simulink model "SM_Regen"  (R2023a)
settings: Solver=ode45  StartTime=0  StopTime=20  FixedStep=0.002  RelTol=1e-3  AbsTol=1e-6
libraries: Solver_SF x1
settings Model: ExtModeTrigMode=oneshot  VariantFading=off  Creator=ywata  LastModifiedBy=USER
settings SolverCC: AutoScaleAbsTol=off  AlgebraicLoopSolver=TrustRegion
settings DataIOCC: SaveFormat=Array  SignalLoggingSaveFormat=ModelDataLogs  ReturnWorkspaceOutputs=off  SignalLoggingName=sigsOut
settings OptimizationCC: BlockReduction=off  BooleanDataType=off  ExpressionDepthLimit=2147483647  LifeSpan=inf
settings DebuggingCC: SaveWithParameterizedLinksMsg=none  UnderspecifiedInitializationDetection=Classic  MergeDetectMultiDrivingBlocksExec=none  SignalResolutionControl=TryResolveAllWithWarning  MultiTaskDSMMsg=warning  MultiTaskCondExecSysMsg=none  FcnCallInpInsideContextMsg=warning  UnconnectedInputMsg=warning  UnconnectedOutputMsg=warning  UnconnectedLineMsg=warning  StateNameClashWarn=warning  SFUnexpectedBacktrackingDiag=warning  SFNoUnconditionalDefaultTransitionDiag=warning  SFExecutionAtInitializationDiag=none  ArithmeticOperatorsInVariantConditions=warning
settings HardwareCC: ProdBitPerPointer=32  ProdBitPerSizeT=32  ProdBitPerPtrDiffT=32  ProdLargestAtomicFloat=None  ProdIntDivRoundTo=Undefined  ProdEndianess=Unspecified  ProdWordSize=32  ProdHWDeviceType=32-bit Generic  TargetUnknown=on
settings ModelReferenceCC: PropagateSignalLabelsOutOfModel=off
settings SFSimCC: SimUseLocalCustomCode=off  CustomCodeUndefinedFunction=UseInterfaceOnly
settings RTWCC: TemplateMakefile=grt_vc.tmf  RTWUseLocalCustomCode=off
settings CodeAppCC: StateflowObjectComments=on
settings GRTTargetCC: TargetFcnLib=ansi_tfl_tmw.mat  TargetLangStandard=C89/C90 (ANSI)  CombineOutputUpdateFcns=off  GRTInterface=on
settings ConfigComp: CovMetricSettings=dw  CovSaveCumulativeToWorkspaceVar=on  CovSaveSingleToWorkspaceVar=on  CovExternalEMLEnable=off

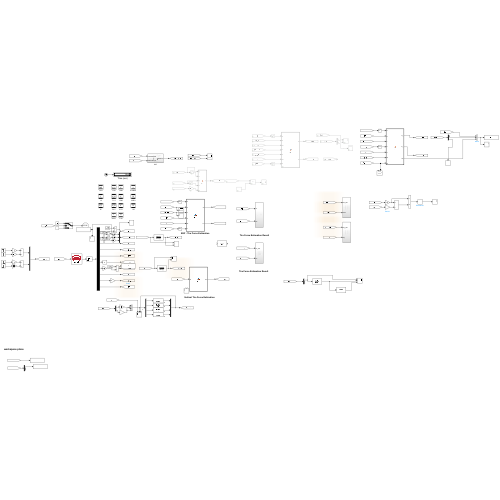
[thumbnail: Simulink's stored preview of the top-level diagram]
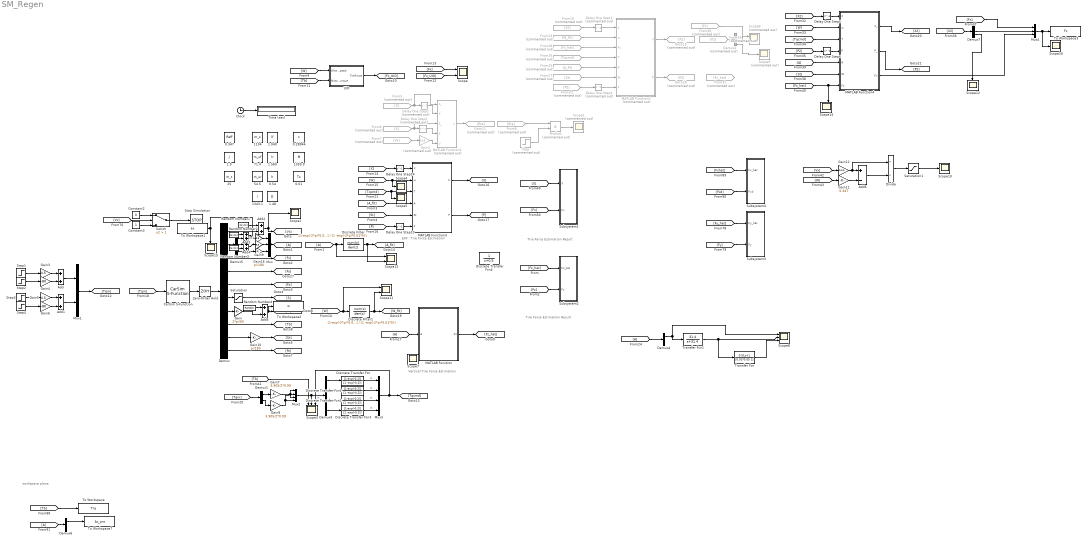
== system SM_Regen ==
  note: workspace place
  note: EKF : Tire Force Estimation
  note: Tire Force Estimation Result
  note: Vertical Tire Force Estimation
  note: Tire Force Estimation Result
  0.01 : DataStoreMemory  DataStoreName=Ts  WriteAfterWriteMsg=warning  InitialValue=0.01  ShowAdditionalParam=off  OutDataTypeStr=double
  0.28944 : DataStoreMemory  DataStoreName=c  WriteAfterWriteMsg=warning  InitialValue=0.29844  ShowAdditionalParam=off  OutDataTypeStr=double
  0.347 : DataStoreMemory  DataStoreName=Reff  WriteAfterWriteMsg=warning  InitialValue=0.347  ShowAdditionalParam=off  OutDataTypeStr=double
  0.54 : DataStoreMemory  DataStoreName=h  WriteAfterWriteMsg=warning  InitialValue=0.54  ShowAdditionalParam=off  OutDataTypeStr=double
  1.040 : DataStoreMemory  DataStoreName=lf  WriteAfterWriteMsg=warning  InitialValue=1.040  ShowAdditionalParam=off  OutDataTypeStr=double
  1.48 : DataStoreMemory  DataStoreName=D  WriteAfterWriteMsg=warning  InitialValue=1.48  ShowAdditionalParam=off  OutDataTypeStr=double
  1.560 : DataStoreMemory  DataStoreName=lr  WriteAfterWriteMsg=warning  InitialValue=1.560  ShowAdditionalParam=off  OutDataTypeStr=double
  1.9 : DataStoreMemory  DataStoreName=J  WriteAfterWriteMsg=warning  InitialValue=1.9  ShowAdditionalParam=off  OutDataTypeStr=double
  1134 : DataStoreMemory  DataStoreName=m_s  WriteAfterWriteMsg=warning  InitialValue=1134  ShowAdditionalParam=off  OutDataTypeStr=double
  1343.1 : DataStoreMemory  DataStoreName=I  WriteAfterWriteMsg=warning  InitialValue=1343.1  ShowAdditionalParam=off  OutDataTypeStr=double
  1359.9 : DataStoreMemory  DataStoreName=M  WriteAfterWriteMsg=warning  InitialValue=1359.9  ShowAdditionalParam=off  OutDataTypeStr=double
  25 : DataStoreMemory  DataStoreName=m_t  WriteAfterWriteMsg=warning  InitialValue=25  ShowAdditionalParam=off  OutDataTypeStr=double
  54.5 : DataStoreMemory  DataStoreName=m_ur  WriteAfterWriteMsg=warning  InitialValue=54.5  ShowAdditionalParam=off  OutDataTypeStr=double
  71.4 : DataStoreMemory  DataStoreName=m_uf  WriteAfterWriteMsg=warning  InitialValue=71.4  ShowAdditionalParam=off  OutDataTypeStr=double
  Add{,1..5} (6 alike) : Sum
  Add6 : Sum  Inputs=+-
  CarSim S-Function : Solver_SF/CarSim S-Function  Priority=1  SIMFILE=simfile.sim  Run_RTs=off  vs_state_ind=Run  StopMode_ind=Vehicle Model
  Clock : Clock
  Constant2 : Constant  Value=0
  Constant3 : Constant
  Delay One Step1 : Delay  Commented=on  DelayLength=1  InitialCondition=[67.655 67.655 67.655 67.655 0 0 0 0 0 0]'  SampleTime=0.01
  Delay One Step10 : Delay  DelayLength=1  InitialCondition=diag([64.1 64.1 64.1 64.1 0 0 0 0])  SampleTime=0.01
  Delay One Step14 : Delay  DelayLength=1  InitialCondition=[64.1 64.1 64.1 64.1 0 0 0 0]'  SampleTime=0.01
  Delay One Step2 : Delay  Commented=on  DelayLength=1  InitialCondition=[0 0 0 0]'  SampleTime=0.01
  Delay One Step3 : Delay  Commented=on  DelayLength=1  InitialCondition=[64.1 64.1 64.1 64.1 0 0 0 0 3930 2740 3930 2740 0]'  SampleTime=0.01
  Delay One Step4 : Delay  Commented=on  DelayLength=1  InitialCondition=diag([64.1 64.1 64.1 64.1 0 0 0 0 3930 2740 3930 2740 0])  SampleTime=0.01
  Delay One Step5 : Delay  DelayLength=1  InitialCondition=[64.1 64.1 64.1 64.1 0 0 0 0 0]'  SampleTime=0.01
  Delay One Step6 : Delay  DelayLength=1  InitialCondition=diag([64.1 64.1 64.1 64.1 0 0 0 0 0])  SampleTime=0.01
  Demux : Demux  Outputs=[1 3 4 4 4 4 4 4 2 2]
  Demux1 : Demux  Outputs=2
  Demux2 : Demux  Commented=on  Outputs=[4 4 4 1]
  Demux3 : Demux
  Demux4 : Demux  Outputs=3
  Demux5 : Demux  Outputs=[1 1 1]
  Demux6 : Demux  Outputs=3
  Demux7 : Demux  Outputs=[4 4 1]
  Discrete Transfer Fcn{,1..3} (4 alike) : DiscreteTransferFcn  Numerator=[1-exp(-0.2)]  Denominator=[1 -exp(-0.2)]
  Discrete Transfer Fcn4 : DiscreteTransferFcn
  Discrete Filter : DiscreteFilter  Numerator=[1-exp(-2*pi*0.01*5)]  Denominator=[1 -exp(-2*pi*0.01*5)]  SampleTime=0.01
  Discrete Filter1 : DiscreteFilter  Numerator=[1-exp(-2*pi*0.01*5)]  Denominator=[1 -exp(-2*pi*0.01*5)]  InitialStates=240  SampleTime=0.01
  Divide : Product  Inputs=/*
  From{1,17,24,39,91} (5 alike) : From
  From19 : From  Commented=on  GotoTag=X2
  From22 : From  Commented=on  GotoTag=P2
  From23 : From  Commented=on  GotoTag=W_flt
  From25 : From  Commented=on  GotoTag=A_flt
  From26 : From  Commented=on  GotoTag=Tqcmd
  From27 : From  Commented=on  GotoTag=St
  From28 : From  Commented=on  GotoTag=Fz_hat
  From29 : From  Commented=on  GotoTag=X2
  From30 : From  Commented=on  GotoTag=Fx
  From31 : From  Commented=on  GotoTag=Fz_hat
  From5 : From  Commented=on  GotoTag=X
  From6 : From  Commented=on  GotoTag=S
  From7 : From  Commented=on  GotoTag=Vx
  From8 : From  Commented=on  GotoTag=Eta
  Gain : Gain  Gain=2*pi/60
  Gain1 : Gain  Gain=9.8
  Gain10 : Gain  Gain=pi/180
  Gain11 : Gain  Gain=0.347
  Gain12 : Gain  Gain=1/3.6
  Gain16 : Gain  Gain=pi/180
  Gain2 : Gain  Commented=on  Gain=1/3.6
  Gain3 : Gain  Gain=4.5
  Gain4 : Gain  Gain=-80
  Gain5 : Gain  Gain=4.5
  Gain6 : Gain  Gain=-80
  Gain7 : Gain  Gain=3.905/2*0.99
  Gain8 : Gain  Gain=3.905/2*0.99
  Gain9 : Gain  Gain=9.8
  Goto1 : Goto
  Goto11 : Goto  Commented=on  GotoTag=Eta
  Goto15 : Goto  Commented=on  GotoTag=X2
  Goto18 : Goto  Commented=on  GotoTag=P2
  MATLAB Function : MATLAB Function  TreatAsAtomicUnit=on
  MATLAB Function1 : MATLAB Function  Commented=on  TreatAsAtomicUnit=on
  MATLAB Function2 : MATLAB Function  Commented=on  TreatAsAtomicUnit=on
  MATLAB Function3 : MATLAB Function  TreatAsAtomicUnit=on
  MATLAB Function4 : MATLAB Function  TreatAsAtomicUnit=on
  Mux : Mux  Inputs=3
  Mux1 : Mux  Inputs=2
  Mux2 : Mux
  Mux3 : Mux
  Mux4 : Mux  Inputs=3
  Product : Product  Commented=on
  Random Number1 : RandomNumber  Variance=0.0005  Seed=2  SampleTime=0.01
  Random Number2 : RandomNumber  Variance=0.0002  Seed=1  SampleTime=0.01
  Random Number3 : RandomNumber  Variance=0.0002  SampleTime=0.01
  Random Number4 : RandomNumber  Variance=0.002  SampleTime=0.01
  Saturation : Saturate  UpperLimit=1  LowerLimit=-1
  Saturation1 : Saturate  UpperLimit=1  LowerLimit=-1
  Scope{,11,13..14} (4 alike) : Scope  NumInputPorts=2
  Scope1 : Scope  Commented=on
  Scope{2,4..5,7,10,12,15..16} (8 alike) : Scope
  Scope3 : Scope  NumInputPorts=3
  Scope6 : Scope  Commented=on  NumInputPorts=2
  Scope8 : Scope  NumInputPorts=3
  Scope9 : Scope  Commented=on
  Step : Step  Commented=on  Time=5  SampleTime=0.01
  Step1 : Step  Time=5  Before=1  After=0  SampleTime=0.01
  Step2 : Step  Time=5  SampleTime=0.01
  Step3 : Step  Time=5  Before=1  After=0  SampleTime=0.01
  Step4 : Step  Time=5  SampleTime=0.01
  Stop Simulation : Stop
  Subsystem1 : Subsystem
  Subsystem2 : Subsystem
  Subsystem3 : Subsystem
  Subsystem4 : Subsystem
  Switch : Switch  Criteria=u2 > Threshold  Threshold=1  SaturateOnIntegerOverflow=off  InputSameDT=off
  Time (sec) : Display
      settings: Format=bank  Decimation=100
  To Workspace : ToWorkspace  VariableName=Trq  SaveFormat=Timeseries  SampleTime=-1
  To Workspace1 : ToWorkspace  VariableName=ax  SaveFormat=Timeseries  SampleTime=-1
  To Workspace2 : ToWorkspace  VariableName=w  SaveFormat=Timeseries  SampleTime=-1
  To Workspace3 : ToWorkspace  VariableName=Fx  SaveFormat=Timeseries  SampleTime=-1
  To Workspace7 : ToWorkspace  VariableName=Ax_pro  SaveFormat=Timeseries  SampleTime=-1
  Transfer Fcn : TransferFcn  Numerator=[0.01 1]  Denominator=[0.01*0.05 1]
  Transfer Fcn1 : TransferFcn  Numerator=[31.4]  Denominator=[1 31.4]
  UIO : Subsystem
  Zero-Order Hold : ZeroOrderHold  SampleTime=0.01
  wires:
  CarSim S-Function/1 -> Zero-Order Hold/1
  Clock/1 -> Time (sec)/1
  Demux/3 -> [Fx]
  Zero-Order Hold/1 -> Demux/1
  Saturation/1 -> [S]
  Demux/2 -> Demux5/1
  Demux5/1 -> Add3/2
  Demux5/3 -> Gain16/1
  Gain1/1 -> Mux/1
  Demux/8 -> [Tb]
  Demux/7 -> Gain/1
  Demux/6 -> Saturation/1
  Demux/5 -> [Fz]
  Demux/4 -> [Fy]
  Gain16/1 -> Mux/3
  [P] -> Delay One Step10/1
  [W] -> Scope4/1, MATLAB Function3/2(w)
  [X] -> Delay One Step14/1
  MATLAB Function3/2(P) -> [P]
  Delay One Step10/1 -> MATLAB Function3/6("P ")
  MATLAB Function3/1(X) -> [X]
  Delay One Step14/1 -> MATLAB Function3/1("X ")
  Gain10/1 -> [St]
  [X] -> Subsystem1/1(X)
  [Fx] -> Subsystem1/2(Fx)
  MATLAB Function/1(Fz) -> [Fz_hat]
  [Fz_hat] -> Subsystem2/1(Fz_hat)
  [Fz] -> Subsystem2/2(Fz)
  [Vx] -> Switch/2
  Constant2/1 -> Switch/1
  Constant3/1 -> Switch/3
  Switch/1 -> Stop Simulation/1
  [Fy] -> Subsystem3/2(Fy)
  [Fy_hat] -> Subsystem3/1(Fy_hat)
  [Tb] -> To Workspace/1
  [Fxd] -> Subsystem4/2(Fxd)
  [Fxhat] -> Subsystem4/1(Fx_hat)
  From91/1 -> Demux6/1
  Demux6/1 -> To Workspace7/1
  [A_flt] -> MATLAB Function3/4(A)
  From5/1 -> MATLAB Function1/1(X_), Delay One Step1/1
  Delay One Step1/1 -> MATLAB Function1/2(X)
  From6/1 -> MATLAB Function1/3(S_), Delay One Step2/1
  Delay One Step2/1 -> MATLAB Function1/4(S)
  From7/1 -> Gain2/1
  [St] -> MATLAB Function3/5(St)
  Gain2/1 -> MATLAB Function1/5(V)
  MATLAB Function1/1(y) -> Goto11/1
  From8/1 -> Product/1
  Step/1 -> Product/2
  Product/1 -> Scope1/1
  Step1/1 -> Gain3/1
  Gain3/1 -> Add/1
  Step2/1 -> Gain4/1
  Gain4/1 -> Add/2
  Add/1 -> Mux1/1
  Add1/1 -> Mux1/2
  Step4/1 -> Gain6/1
  Gain6/1 -> Add1/2
  Gain5/1 -> Add1/1
  Step3/1 -> Gain5/1
  Mux1/1 -> [Tqin]
  Add3/1 -> To Workspace1/1, Scope15/1, Gain1/1
  Gain/1 -> Add5/2
  Random Number4/1 -> Add5/1
  Add5/1 -> To Workspace2/1, [W]
  Demux/9 -> Gain10/1
  Demux/10 -> [Pc]
  Demux/1 -> Add2/2
  Add2/1 -> Scope2/1, [Vx]
  Random Number1/1 -> Add2/1
  [W] -> UIO/1(WheelSpeed)
  [Tb] -> UIO/2(MotorTorque)
  UIO/1(TireForce) -> [Fx_UIO]
  [Fx_UIO] -> Scope/2
  [Fx] -> Scope/1
  [Tqin] -> CarSim S-Function/1
  [Tqin] -> Demux1/1
  Demux1/1 -> Gain7/1
  Demux1/2 -> Gain8/1
  Gain7/1 -> Mux2/1, Mux2/3
  Gain8/1 -> Mux2/4, Mux2/2
  Mux2/1 -> Demux3/1, Scope3/2  "in"
  Demux3/1 -> Discrete Transfer Fcn/1
  Discrete Transfer Fcn/1 -> Mux3/1  "in"
  Demux3/4 -> Discrete Transfer Fcn3/1
  Demux3/3 -> Discrete Transfer Fcn2/1
  Demux3/2 -> Discrete Transfer Fcn1/1
  Discrete Transfer Fcn2/1 -> Mux3/3  "in"
  Discrete Transfer Fcn1/1 -> Mux3/2  "in"
  Discrete Transfer Fcn3/1 -> Mux3/4  "in"
  Mux3/1 -> [Tqcmd], Scope3/3
  [Tqcmd] -> Scope5/1, MATLAB Function3/3(T)
  Mux/1 -> Goto1/1
  Random Number3/1 -> Add4/2
  Demux5/2 -> Add4/1
  Add4/1 -> Gain9/1
  Gain9/1 -> Mux/2
  Random Number2/1 -> Add3/1
  From1/1 -> Scope13/1, Discrete Filter/1
  Discrete Filter/1 -> Scope13/2, [A_flt]
  From17/1 -> MATLAB Function/1(A)
  MATLAB Function2/1(X) -> Goto15/1
  MATLAB Function2/2(P) -> Goto18/1
  From23/1 -> MATLAB Function2/2(w)
  Transfer Fcn1/1 -> Scope8/2, Transfer Fcn/1
  Transfer Fcn/1 -> Scope8/3
  Demux4/1 -> Scope8/1, Transfer Fcn1/1
  From24/1 -> Demux4/1
  [W] -> Scope11/1, Discrete Filter1/1
  Discrete Filter1/1 -> Scope11/2, [W_flt]
  From25/1 -> MATLAB Function2/5(A)
  From27/1 -> MATLAB Function2/6(St)
  From26/1 -> MATLAB Function2/4(T)
  From19/1 -> Delay One Step3/1
  Delay One Step3/1 -> MATLAB Function2/1("X ")
  From22/1 -> Delay One Step4/1
  Delay One Step4/1 -> MATLAB Function2/7("P ")
  From28/1 -> MATLAB Function2/3(Fz)
  From29/1 -> Demux2/1
  Demux2/4 -> Scope9/1
  Demux2/2 -> Scope6/2
  From30/1 -> Scope6/1
  [X2] -> Delay One Step5/1
  MATLAB Function4/1(X_) -> [X2]
  Delay One Step5/1 -> MATLAB Function4/1(X)
  [W] -> MATLAB Function4/2(w)
  [Tqcmd] -> MATLAB Function4/3(T)
  MATLAB Function4/2(P_) -> [P2]
  [P2] -> Delay One Step6/1
  Delay One Step6/1 -> MATLAB Function4/4(P)
  [X2] -> Demux7/1
  Demux7/2 -> Mux4/2
  [Fx] -> Mux4/1
  [St] -> MATLAB Function4/6(St)
  From39/1 -> MATLAB Function4/5(A)
  Demux7/3 -> Scope12/1
  [Fz_hat] -> Scope14/2, MATLAB Function4/7(Fz)
  MATLAB Function4/3(Fx) -> Mux4/3
  [Tb] -> Scope3/1
  Mux4/1 -> Scope16/1, To Workspace3/1
  [Vx] -> Gain12/1
  [W] -> Gain11/1
  Add6/1 -> Divide/2
  Divide/1 -> Saturation1/1
  Gain12/1 -> Divide/1, Add6/1
  Gain11/1 -> Add6/2
  Saturation1/1 -> Scope10/1

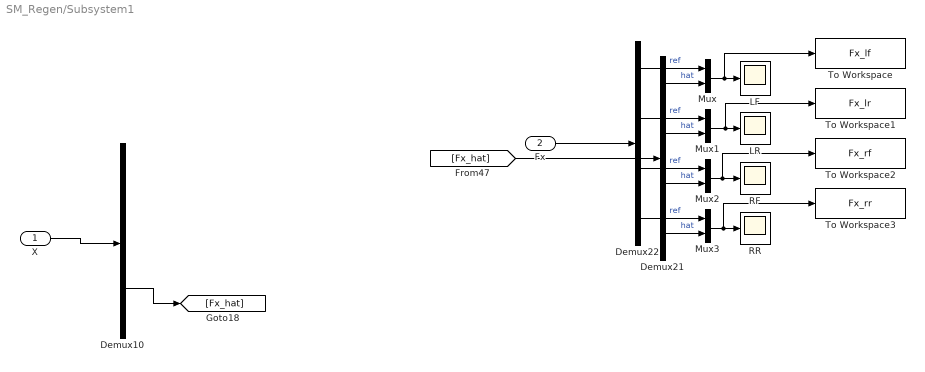
== system SM_Regen/Subsystem1 ==
  X : Inport
  Fx : Inport  Port=2
  Demux10 : Demux  Outputs=[4 4]
  Demux21 : Demux
  Demux22 : Demux
  LF : Scope
  LR : Scope
  Mux{,1..3} (4 alike) : Mux  Inputs=2
  RF : Scope
  RR : Scope
  To Workspace : ToWorkspace  VariableName=Fx_lf  SaveFormat=Timeseries  SampleTime=-1
  To Workspace1 : ToWorkspace  VariableName=Fx_lr  SaveFormat=Timeseries  SampleTime=-1
  To Workspace2 : ToWorkspace  VariableName=Fx_rf  SaveFormat=Timeseries  SampleTime=-1
  To Workspace3 : ToWorkspace  VariableName=Fx_rr  SaveFormat=Timeseries  SampleTime=-1
  wires:
  Demux21/3 -> Mux2/2  "hat"
  [Fx_hat] -> Demux21/1
  Demux21/4 -> Mux3/2  "hat"
  Fx/1 -> Demux22/1
  Demux22/4 -> Mux3/1  "ref"
  Demux21/1 -> Mux/2  "hat"
  Demux22/3 -> Mux2/1  "ref"
  Demux22/2 -> Mux1/1  "ref"
  Demux21/2 -> Mux1/2  "hat"
  X/1 -> Demux10/1
  Demux10/2 -> [Fx_hat]
  Demux22/1 -> Mux/1  "ref"
  Mux/1 -> To Workspace/1, LF/1
  Mux1/1 -> To Workspace1/1, LR/1
  Mux2/1 -> To Workspace2/1, RF/1
  Mux3/1 -> To Workspace3/1, RR/1

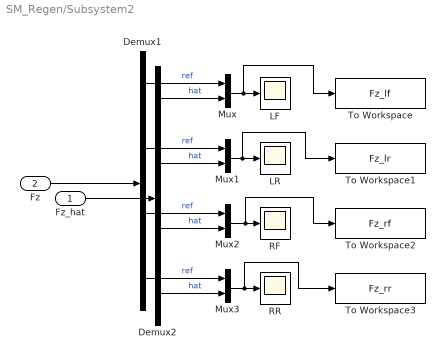
== system SM_Regen/Subsystem2 ==
  Fz_hat : Inport
  Fz : Inport  Port=2
  Demux1 : Demux
  Demux2 : Demux
  LF : Scope
  LR : Scope
  Mux{,1..3} (4 alike) : Mux  Inputs=2
  RF : Scope
  RR : Scope
  To Workspace : ToWorkspace  VariableName=Fz_lf  SaveFormat=Timeseries  SampleTime=-1
  To Workspace1 : ToWorkspace  VariableName=Fz_lr  SaveFormat=Timeseries  SampleTime=-1
  To Workspace2 : ToWorkspace  VariableName=Fz_rf  SaveFormat=Timeseries  SampleTime=-1
  To Workspace3 : ToWorkspace  VariableName=Fz_rr  SaveFormat=Timeseries  SampleTime=-1
  wires:
  Fz_hat/1 -> Demux2/1
  Fz/1 -> Demux1/1
  Demux1/1 -> Mux/1  "ref"
  Demux2/1 -> Mux/2  "hat"
  Demux2/2 -> Mux1/2  "hat"
  Demux1/2 -> Mux1/1  "ref"
  Demux1/3 -> Mux2/1  "ref"
  Demux2/3 -> Mux2/2  "hat"
  Demux1/4 -> Mux3/1  "ref"
  Demux2/4 -> Mux3/2  "hat"
  Mux/1 -> To Workspace/1, LF/1
  Mux1/1 -> To Workspace1/1, LR/1
  Mux2/1 -> To Workspace2/1, RF/1
  Mux3/1 -> To Workspace3/1, RR/1

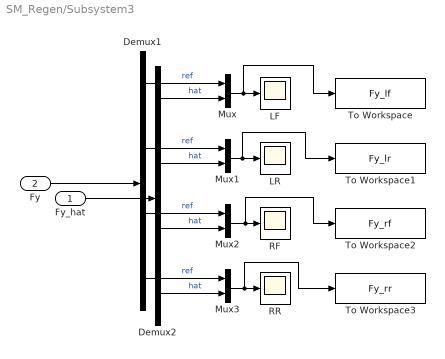
== system SM_Regen/Subsystem3 ==
  Fy_hat : Inport
  Fy : Inport  Port=2
  Demux1 : Demux
  Demux2 : Demux
  LF : Scope
  LR : Scope
  Mux{,1..3} (4 alike) : Mux  Inputs=2
  RF : Scope
  RR : Scope
  To Workspace : ToWorkspace  VariableName=Fy_lf  SaveFormat=Timeseries  SampleTime=-1
  To Workspace1 : ToWorkspace  VariableName=Fy_lr  SaveFormat=Timeseries  SampleTime=-1
  To Workspace2 : ToWorkspace  VariableName=Fy_rf  SaveFormat=Timeseries  SampleTime=-1
  To Workspace3 : ToWorkspace  VariableName=Fy_rr  SaveFormat=Timeseries  SampleTime=-1
  wires:
  Fy_hat/1 -> Demux2/1
  Fy/1 -> Demux1/1
  Demux1/1 -> Mux/1  "ref"
  Demux2/1 -> Mux/2  "hat"
  Demux2/2 -> Mux1/2  "hat"
  Demux1/2 -> Mux1/1  "ref"
  Demux1/3 -> Mux2/1  "ref"
  Demux2/3 -> Mux2/2  "hat"
  Demux1/4 -> Mux3/1  "ref"
  Demux2/4 -> Mux3/2  "hat"
  Mux/1 -> To Workspace/1, LF/1
  Mux1/1 -> To Workspace1/1, LR/1
  Mux2/1 -> To Workspace2/1, RF/1
  Mux3/1 -> To Workspace3/1, RR/1

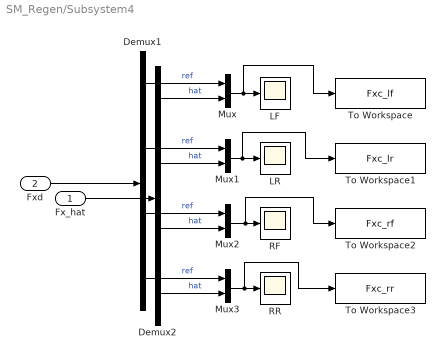
== system SM_Regen/Subsystem4 ==
  Fx_hat : Inport
  Fxd : Inport  Port=2
  Demux1 : Demux
  Demux2 : Demux
  LF : Scope
  LR : Scope
  Mux{,1..3} (4 alike) : Mux  Inputs=2
  RF : Scope
  RR : Scope
  To Workspace : ToWorkspace  VariableName=Fxc_lf  SaveFormat=Timeseries  SampleTime=-1
  To Workspace1 : ToWorkspace  VariableName=Fxc_lr  SaveFormat=Timeseries  SampleTime=-1
  To Workspace2 : ToWorkspace  VariableName=Fxc_rf  SaveFormat=Timeseries  SampleTime=-1
  To Workspace3 : ToWorkspace  VariableName=Fxc_rr  SaveFormat=Timeseries  SampleTime=-1
  wires:
  Fx_hat/1 -> Demux2/1
  Fxd/1 -> Demux1/1
  Demux1/1 -> Mux/1  "ref"
  Demux2/1 -> Mux/2  "hat"
  Demux2/2 -> Mux1/2  "hat"
  Demux1/2 -> Mux1/1  "ref"
  Demux1/3 -> Mux2/1  "ref"
  Demux2/3 -> Mux2/2  "hat"
  Demux1/4 -> Mux3/1  "ref"
  Demux2/4 -> Mux3/2  "hat"
  Mux/1 -> To Workspace/1, LF/1
  Mux1/1 -> To Workspace1/1, LR/1
  Mux2/1 -> To Workspace2/1, RF/1
  Mux3/1 -> To Workspace3/1, RR/1

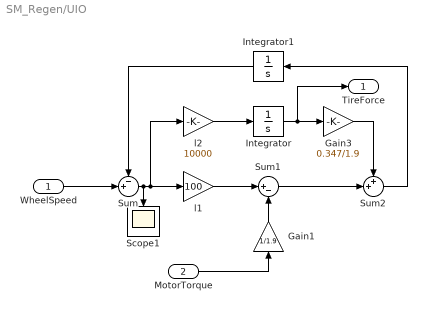
== system SM_Regen/UIO ==
  WheelSpeed : Inport
  MotorTorque : Inport  Port=2
  Gain1 : Gain  Gain=1/1.9
  Gain3 : Gain  Gain=0.347/1.9
  Integrator : Integrator  InitialCondition=[0 0 0 0]'
  Integrator1 : Integrator  InitialCondition=[64.1 64.1 64.1 64.1]'
  Scope1 : Scope
  Sum : Sum  Inputs=-+|
  Sum1 : Sum  Inputs=|+-
  Sum2 : Sum  Inputs=++|
  l1 : Gain  Gain=100
  l2 : Gain  Gain=10000
  TireForce : Outport
  wires:
  WheelSpeed/1 -> Sum/2
  Sum/1 -> Scope1/1, l2/1, l1/1
  MotorTorque/1 -> Gain1/1
  l1/1 -> Sum1/1
  Gain1/1 -> Sum1/2
  l2/1 -> Integrator/1
  Integrator/1 -> TireForce/1, Gain3/1
  Sum1/1 -> Sum2/2
  Gain3/1 -> Sum2/1
  Sum2/1 -> Integrator1/1
  Integrator1/1 -> Sum/1

== matlab function SM_Regen/MATLAB Function4 ==
  data: X input; w input; T input; X_ output; P_ output; P input; Reff data_store_memory; J data_store_memory; Ts data_store_memory; I data_store_memory; M data_store_memory; lf data_store_memory; lr data_store_memory; D data_store_memory; A input; St input; Fz input; Fx output
function [X_,P_,Fx]  = fcn(X,w,T,P,A,St,Fz)

global  Reff J Ts M;

%X = [w_lf w_lr w_rf w_rr F_lf F_lr F_rf F_rr Crr]
Q = diag([0.0001 0.0001 0.0001 0.0001 10 10 10 10 0.0000001]);

%Z = [w_lf w_lr w_rf w_rr ax]
Z = [w(1),w(2),w(3),w(4),A(1)]';
R = diag([0.002 0.002 0.002 0.002 0.1]);

U = [T(1) T(2)]';
G = [1/J 0;0 1/J;1/J 0;0 1/J;0 0;0 0;0 0;0 0;0 0];

F = eye(9) + Ts*...
    [0 0 0 0 -Reff/J 0 0 0 0;
     0 0 0 0 0 -Reff/J 0 0 0;
     0 0 0 0 0 0 -Reff/J 0 0;
     0 0 0 0 0 0 0 -Reff/J 0;
     zeros(5,9)];

H = [1 0 0 0 0 0 0 0 0;
     0 1 0 0 0 0 0 0 0;
     0 0 1 0 0 0 0 0 0;
     0 0 0 1 0 0 0 0 0;
     0 0 0 0 1/M 1/M 1/M 1/M -9.8];

Xm = F*X + G*U*Ts;
Pm = F*P*F'+Q;
K = Pm*H'/(H*Pm*H'+R);
X_ = Xm+K*(Z-H*Xm);
P_ = (eye(9)-K*H)*Pm;

if abs(St(1)) > pi/180 && abs(St(2)) > pi/180
X_(9) = X(9);
end

Rr = X_(9)*Fz;
Fx = X_(5:8)-Rr;

% Fx = cos(St(1))*X(5)+X(6)+cos(St(2))*X(7)+X(8);
% 
% Crr = (Fx/M-A(1))/9.8;

== matlab function SM_Regen/MATLAB Function1 ==
  data: X_ input; X input; S_ input; S input; y output; V input; Reff data_store_memory
function y = fcn(X_,X,S_,S,V)

global Reff

dX = X-X_;
dS = S-S_;

eta_lf = dX(7)/dS(1);
eta_lr = dX(8)/dS(2);
eta_rf = dX(9)/dS(3);
eta_rr = dX(10)/dS(4);

y = [eta_lf;eta_lr;eta_rf;eta_rr];

== matlab function SM_Regen/MATLAB Function ==
  data: A input; Fz output; m_s data_store_memory; m_uf data_store_memory; m_ur data_store_memory; lf data_store_memory; lr data_store_memory; h data_store_memory; m_t data_store_memory; D data_store_memory
function Fz = fcn(A)

a = [9.8 A(1) A(2)]';

global m_s m_uf m_ur lf lr h m_t D

L = lf+lr;
Mz = [lr/(2*L)*m_s+1/2*m_uf+m_t -h/(2*L)*m_s -h/(2*D)*m_s;
     lf/(2*L)*m_s+1/2*m_ur+m_t h/(2*L)*m_s -h/(2*D)*m_s;
     lr/(2*L)*m_s+1/2*m_uf+m_t -h/(2*L)*m_s h/(2*D)*m_s;
     lf/(2*L)*m_s+1/2*m_ur+m_t h/(2*L)*m_s h/(2*D)*m_s];

Fz = Mz*a;

== matlab function SM_Regen/MATLAB Function3 ==
  data: X input; w input; T input; A input; St input; X output; P output; P input; Reff data_store_memory; J data_store_memory; Ts data_store_memory; I data_store_memory; M data_store_memory; lf data_store_memory; lr data_store_memory; D data_store_memory
function [X,P]  = fcn(X,w,T,A,St,P)

global  Reff J Ts M;

%X = [w_lf w_lr w_rf w_rr F_lf F_lr F_rf F_rr]
Q = diag([0.0001 0.0001 0.0001 0.0001 10 10 10 10]);

%Z = [w_lf w_lr w_rf w_rr ax]
Z = [w(1),w(2),w(3),w(4),A(1)]';
R = diag([0.0002 0.0002 0.0002 0.0002 0.02]);

U = [T(1) T(2)]';
G = [1/J 0;0 1/J;1/J 0;0 1/J;0 0;0 0;0 0;0 0];

F = eye(8) + Ts*...
    [0 0 0 0 -Reff/J 0 0 0;
     0 0 0 0 0 -Reff/J 0 0;
     0 0 0 0 0 0 -Reff/J 0;
     0 0 0 0 0 0 0 -Reff/J;
     zeros(4,8)];

H = [1 0 0 0 0 0 0 0;
     0 1 0 0 0 0 0 0;
     0 0 1 0 0 0 0 0;
     0 0 0 1 0 0 0 0;
     0 0 0 0 cos(St(1))/M 1/M cos(St(2))/M 1/M];

Xm = F*X + G*U*Ts;
Pm = F*P*F'+Q;
K = Pm*H'/(H*Pm*H'+R);
X = Xm+K*(Z-H*Xm);
P = (eye(8)-K*H)*Pm;

end

== matlab function SM_Regen/MATLAB Function2 ==
  data: X input; w input; Fz input; T input; A input; St input; X output; P output; P input; Reff data_store_memory; J data_store_memory; Ts data_store_memory; I data_store_memory; M data_store_memory; lf data_store_memory; lr data_store_memory; D data_store_memory
function [X,P]  = fcn(X,w,Fz,T,A,St,P)

global  Reff J Ts M;

%X = [w_lf w_lr w_rf w_rr Fx_lf Fx_lr Fx_rf Fx_rr Fz_lf Fz_lr Fz_rf Fz_rr Crr]
Q = diag([0.001 0.001 0.001 0.001 10 10 10 10 10 10 10 10 0.00001]);

%Z = [w_lf w_lr w_rf w_rr ax]
Z = [w(1),w(2),w(3),w(4),Fz(1),Fz(2),Fz(3),Fz(4),A(1)]';
R = diag([0.0002 0.0002 0.0002 0.0002 0.05 0.05 0.05 0.05 0.02]);

U = [T(1) T(2)]';
G = [1/J 0;0 1/J;1/J 0;0 1/J;0 0;0 0;0 0;0 0;0 0;0 0;0 0;0 0;0 0];

F = eye(13) + Ts*...
    [0 0 0 0 -Reff/J 0 0 0 -Reff/J*X(13) 0 0 0 -Reff/J*X(9);
     0 0 0 0 0 -Reff/J 0 0 0 -Reff/J*X(13) 0 0 -Reff/J*X(10);
     0 0 0 0 0 0 -Reff/J 0 0 0 -Reff/J*X(13) 0 -Reff/J*X(11);
     0 0 0 0 0 0 0 -Reff/J 0 0 0 -Reff/J*X(13) -Reff/J*X(12);
     zeros(9,13)];

H = [1 0 0 0 0 0 0 0 0 0 0 0 0;
     0 1 0 0 0 0 0 0 0 0 0 0 0;
     0 0 1 0 0 0 0 0 0 0 0 0 0;
     0 0 0 1 0 0 0 0 0 0 0 0 0;
     0 0 0 0 0 0 0 0 1 0 0 0 0;
     0 0 0 0 0 0 0 0 0 1 0 0 0;
     0 0 0 0 0 0 0 0 0 0 1 0 0;
     0 0 0 0 0 0 0 0 0 0 0 1 0;
     0 0 0 0 cos(St(1))/M 1/M cos(St(2))/M 1/M 0 0 0 0 0];

X(1) = X(1) + (-Reff/J*(X(5)+X(9)*X(13))+1/J*U(1))*Ts;
X(2) = X(2) + (-Reff/J*(X(6)+X(10)*X(13))+1/J*U(2))*Ts;
X(3) = X(3) + (-Reff/J*(X(7)+X(11)*X(13))+1/J*U(1))*Ts;
X(4) = X(4) + (-Reff/J*(X(8)+X(12)*X(13))+1/J*U(2))*Ts;
Xm = X;
Pm = F*P*F'+Q;
K = Pm*H'/(H*Pm*H'+R);
X = Xm+K*(Z-H*Xm);
P = (eye(13)-K*H)*Pm;

end
